simulink model "Simluation"  (R2017b)
settings: Solver=VariableStepAuto  StartTime=0.0  StopTime=5  RelTol=1e-3
settings Model: Creator=ASUS  LastModifiedBy=ASUS

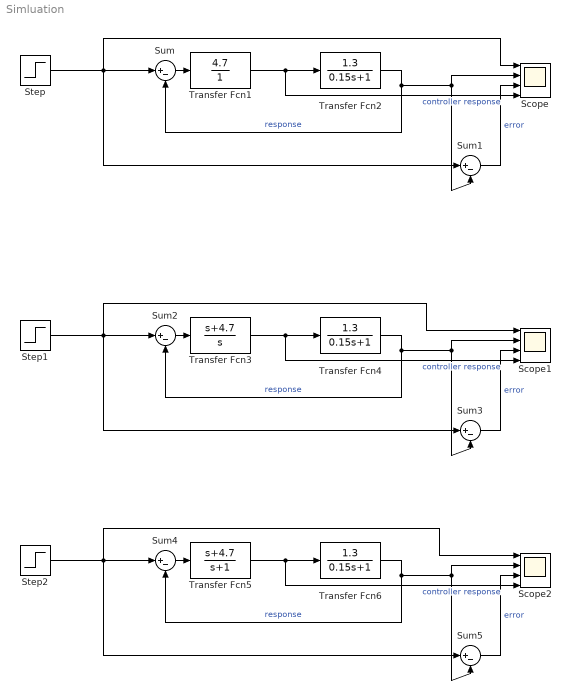
== system Simluation ==
  Scope : Scope  NumInputPorts=4
  Scope1 : Scope  NumInputPorts=4
  Scope2 : Scope  NumInputPorts=4
  Step : Step  SampleTime=0
  Step1 : Step  SampleTime=0
  Step2 : Step  SampleTime=0
  Sum{,1..5} (6 alike) : Sum  Inputs=|+-
  Transfer Fcn1 : TransferFcn  Numerator=[4.7]  Denominator=[1]
  Transfer Fcn2 : TransferFcn  Numerator=[1.3]  Denominator=[0.15 1]
  Transfer Fcn3 : TransferFcn  Numerator=[1 4.7]  Denominator=[1 0]
  Transfer Fcn4 : TransferFcn  Numerator=[1.3]  Denominator=[0.15 1]
  Transfer Fcn5 : TransferFcn  Numerator=[1 4.7]  Denominator=[1 1]
  Transfer Fcn6 : TransferFcn  Numerator=[1.3]  Denominator=[0.15 1]
  wires:
  Transfer Fcn2/1 -> Sum1/2, Scope/2, Sum/2  "response"
  Sum/1 -> Transfer Fcn1/1
  Step/1 -> Sum1/1, Sum/1, Scope/1
  Sum1/1 -> Scope/3  "error"
  Transfer Fcn4/1 -> Sum3/2, Scope1/2, Sum2/2  "response"
  Sum3/1 -> Scope1/3  "error"
  Step1/1 -> Sum3/1, Sum2/1, Scope1/1
  Sum2/1 -> Transfer Fcn3/1
  Transfer Fcn6/1 -> Sum5/2, Scope2/2, Sum4/2  "response"
  Sum5/1 -> Scope2/3  "error"
  Step2/1 -> Sum5/1, Sum4/1, Scope2/1
  Sum4/1 -> Transfer Fcn5/1
  Transfer Fcn3/1 -> Transfer Fcn4/1, Scope1/4  "controller response"
  Transfer Fcn1/1 -> Transfer Fcn2/1, Scope/4  "controller response"
  Transfer Fcn5/1 -> Transfer Fcn6/1, Scope2/4  "controller response"
